simulink model "cas"  (R2019a)
settings: Solver=VariableStepAuto  StartTime=0.0  StopTime=200  RelTol=1e-3
settings Model: Creator=Lenovo  LastModifiedBy=shaosimin
settings DataIOCC: ReturnWorkspaceOutputs=off
settings DebuggingCC: ArithmeticOperatorsInVariantConditions=warning
settings SFSimCC: SimUseLocalCustomCode=off
settings RTWCC: RTWUseLocalCustomCode=off
settings CodeAppCC: StateflowObjectComments=on

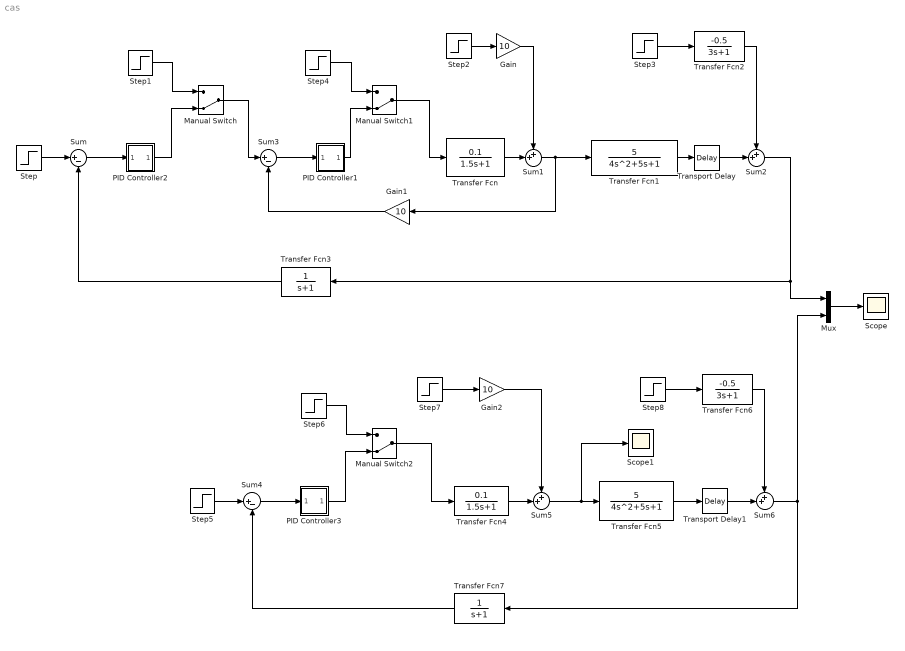
== system cas ==
  Gain : Gain  Gain=10
  Gain1 : Gain  Gain=10
  Gain2 : Gain  Gain=10
  Manual Switch : ManualSwitch  CurrentSetting=0
  Manual Switch1 : ManualSwitch  CurrentSetting=0
  Manual Switch2 : ManualSwitch  CurrentSetting=0
  Mux : Mux  Inputs=2
  PID Controller1 : Subsystem  AncestorBlock=simulink_extras/Additional Linear/PID Controller  mask(PID Controller){P=4, I=1.5, D=0}
      mask prompts: P "Proportional:"; I "Integral:"; D "Derivative:"
      mask help:
      | Enter expressions for proportional, integral, and derivative terms.
      | P+I/s+Ds
      mask Help: This block implements a PID controller where parameters are entered for the Proportional, Integral and Derivative terms. Unmask this block to see how it works. The derivative term is implemented using a true derivative block.
      mask Display: disp('PID')
  PID Controller2 : Subsystem  AncestorBlock=simulink_extras/Additional Linear/PID Controller  mask(PID Controller){P=2.46, I=8.5, D=2.125}
      mask prompts: P "Proportional:"; I "Integral:"; D "Derivative:"
      mask help:
      | Enter expressions for proportional, integral, and derivative terms.
      | P+I/s+Ds
      mask Help: This block implements a PID controller where parameters are entered for the Proportional, Integral and Derivative terms. Unmask this block to see how it works. The derivative term is implemented using a true derivative block.
      mask Display: disp('PID')
  PID Controller3 : Subsystem  AncestorBlock=simulink_extras/Additional Linear/PID Controller  mask(PID Controller){P=2.4, I=9.9, D=2.475}
      mask prompts: P "Proportional:"; I "Integral:"; D "Derivative:"
      mask help:
      | Enter expressions for proportional, integral, and derivative terms.
      | P+I/s+Ds
      mask Help: This block implements a PID controller where parameters are entered for the Proportional, Integral and Derivative terms. Unmask this block to see how it works. The derivative term is implemented using a true derivative block.
      mask Display: disp('PID')
  Scope : Scope
  Scope1 : Scope
  Step{,1,4..6} (5 alike) : Step  Time=0  SampleTime=0
  Step2 : Step  Time=70  After=0.1  SampleTime=0
  Step3 : Step  Time=160  SampleTime=0
  Step7 : Step  Time=70  After=0.1  SampleTime=0
  Step8 : Step  Time=160  SampleTime=0
  Sum : Sum  Inputs=|+-
  Sum{1..2,5..6} (4 alike) : Sum  Inputs=++|
  Sum3 : Sum  Inputs=|+-
  Sum4 : Sum  Inputs=|+-
  Transfer Fcn : TransferFcn  Numerator=[0.1]  Denominator=[1.5 1]
  Transfer Fcn1 : TransferFcn  Numerator=[5]  Denominator=[4 5 1]
  Transfer Fcn2 : TransferFcn  Numerator=[-0.5]  Denominator=[3 1]
  Transfer Fcn3 : TransferFcn  Denominator=[1 1]
  Transfer Fcn4 : TransferFcn  Numerator=[0.1]  Denominator=[1.5 1]
  Transfer Fcn5 : TransferFcn  Numerator=[5]  Denominator=[4 5 1]
  Transfer Fcn6 : TransferFcn  Numerator=[-0.5]  Denominator=[3 1]
  Transfer Fcn7 : TransferFcn  Denominator=[1 1]
  Transport Delay : TransportDelay  DelayTime=3
  Transport Delay1 : TransportDelay  DelayTime=3
  wires:
  Step/1 -> Sum/1
  Sum/1 -> PID Controller2/1(In_1)
  PID Controller2/1(Out_1) -> Manual Switch/2
  Step1/1 -> Manual Switch/1
  Transfer Fcn/1 -> Sum1/2
  Step2/1 -> Gain/1
  Gain/1 -> Sum1/1
  Sum1/1 -> Gain1/1, Transfer Fcn1/1
  Transfer Fcn1/1 -> Transport Delay/1
  Transport Delay/1 -> Sum2/2
  Step3/1 -> Transfer Fcn2/1
  Transfer Fcn2/1 -> Sum2/1
  Sum2/1 -> Mux/1, Transfer Fcn3/1
  Transfer Fcn3/1 -> Sum/2
  Manual Switch/1 -> Sum3/1
  Sum3/1 -> PID Controller1/1(In_1)
  Step4/1 -> Manual Switch1/1
  PID Controller1/1(Out_1) -> Manual Switch1/2
  Manual Switch1/1 -> Transfer Fcn/1
  Gain1/1 -> Sum3/2
  Step5/1 -> Sum4/1
  Sum4/1 -> PID Controller3/1(In_1)
  PID Controller3/1(Out_1) -> Manual Switch2/2
  Step6/1 -> Manual Switch2/1
  Manual Switch2/1 -> Transfer Fcn4/1
  Transfer Fcn4/1 -> Sum5/2
  Step7/1 -> Gain2/1
  Gain2/1 -> Sum5/1
  Sum5/1 -> Scope1/1, Transfer Fcn5/1
  Transfer Fcn5/1 -> Transport Delay1/1
  Transport Delay1/1 -> Sum6/2
  Step8/1 -> Transfer Fcn6/1
  Transfer Fcn6/1 -> Sum6/1
  Sum6/1 -> Mux/2, Transfer Fcn7/1
  Transfer Fcn7/1 -> Sum4/2
  Mux/1 -> Scope/1

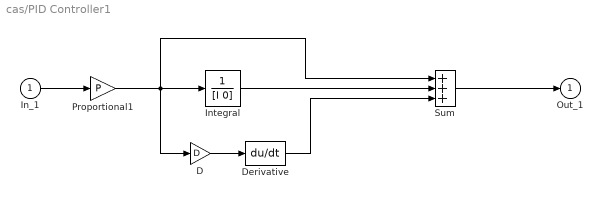
== system cas/PID Controller1 ==
  In_1 : Inport
  D : Gain  Gain=D  SaturateOnIntegerOverflow=on  OutDataTypeStr=Inherit: Same as input  ParamDataTypeStr=Inherit: Same as input
  Derivative : Derivative
  Integral : TransferFcn  Denominator=[I 0]
  Proportional1 : Gain  Gain=P  SaturateOnIntegerOverflow=on  OutDataTypeStr=Inherit: Same as input  ParamDataTypeStr=Inherit: Same as input
  Sum : Sum  Inputs=+++  SaturateOnIntegerOverflow=on  InputSameDT=on  OutDataTypeStr=Inherit: Same as first input
  Out_1 : Outport  InitialOutput=0
  wires:
  Proportional1/1 -> Sum/1, D/1, Integral/1
  Integral/1 -> Sum/2
  Derivative/1 -> Sum/3
  Sum/1 -> Out_1/1
  D/1 -> Derivative/1
  In_1/1 -> Proportional1/1

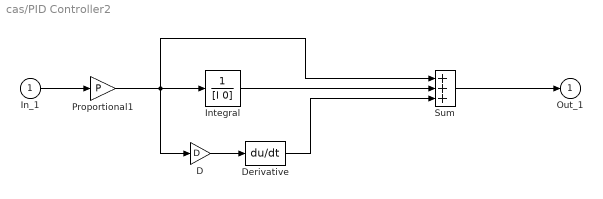
== system cas/PID Controller2 ==
  In_1 : Inport
  D : Gain  Gain=D  SaturateOnIntegerOverflow=on  OutDataTypeStr=Inherit: Same as input  ParamDataTypeStr=Inherit: Same as input
  Derivative : Derivative
  Integral : TransferFcn  Denominator=[I 0]
  Proportional1 : Gain  Gain=P  SaturateOnIntegerOverflow=on  OutDataTypeStr=Inherit: Same as input  ParamDataTypeStr=Inherit: Same as input
  Sum : Sum  Inputs=+++  SaturateOnIntegerOverflow=on  InputSameDT=on  OutDataTypeStr=Inherit: Same as first input
  Out_1 : Outport  InitialOutput=0
  wires:
  Proportional1/1 -> Sum/1, D/1, Integral/1
  Integral/1 -> Sum/2
  Derivative/1 -> Sum/3
  Sum/1 -> Out_1/1
  D/1 -> Derivative/1
  In_1/1 -> Proportional1/1

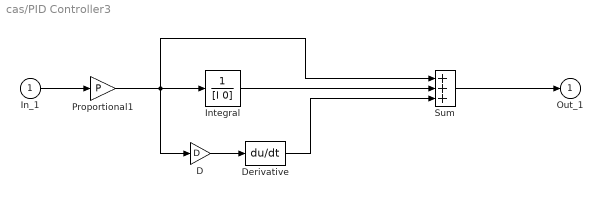
== system cas/PID Controller3 ==
  In_1 : Inport
  D : Gain  Gain=D  SaturateOnIntegerOverflow=on  OutDataTypeStr=Inherit: Same as input  ParamDataTypeStr=Inherit: Same as input
  Derivative : Derivative
  Integral : TransferFcn  Denominator=[I 0]
  Proportional1 : Gain  Gain=P  SaturateOnIntegerOverflow=on  OutDataTypeStr=Inherit: Same as input  ParamDataTypeStr=Inherit: Same as input
  Sum : Sum  Inputs=+++  SaturateOnIntegerOverflow=on  InputSameDT=on  OutDataTypeStr=Inherit: Same as first input
  Out_1 : Outport  InitialOutput=0
  wires:
  Proportional1/1 -> Sum/1, D/1, Integral/1
  Integral/1 -> Sum/2
  Derivative/1 -> Sum/3
  Sum/1 -> Out_1/1
  D/1 -> Derivative/1
  In_1/1 -> Proportional1/1
